simulink model "tarmodel"  (R2019b)
settings: Solver=ode3  StartTime=0.0  StopTime=10.0  RelTol=1e-3
Description:
  | ###CmwHarnessModel###
settings Model: Creator=chin.j  LastModifiedBy=user4.gaio
settings DataIOCC: SaveOutput=off  SaveTime=off  ReturnWorkspaceOutputs=off
settings OptimizationCC: LifeSpan=inf
settings DebuggingCC: StrictBusMsg=ErrorOnBusTreatedAsVector  SFExecutionAtInitializationDiag=none  ArithmeticOperatorsInVariantConditions=warning
settings HardwareCC: ProdBitPerSizeT=32  ProdBitPerPtrDiffT=32  ProdWordSize=32  ProdHWDeviceType=Specified
settings SFSimCC: CustomCodeUndefinedFunction=UseInterfaceOnly
settings CodeAppCC: StateflowObjectComments=on

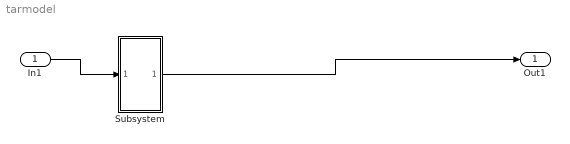
== system tarmodel ==
  In1 : Inport  OutDataTypeStr=uint8  PortDimensions=1  Interpolate=off
  Subsystem : Subsystem
  Out1 : Outport  OutDataTypeStr=fixdt('ufix16_En4')
  wires:
  In1/1 -> Subsystem/1(In1)
  Subsystem/1(Out1) -> Out1/1

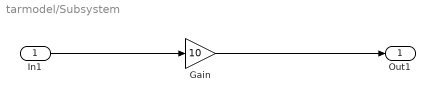
== system tarmodel/Subsystem ==
  In1 : Inport  OutDataTypeStr=uint8
  Gain : Gain  Gain=10
  Out1 : Outport
  wires:
  In1/1 -> Gain/1
  Gain/1 -> Out1/1
